simulink model "simulink2stopnie"  (R2024b)
settings: Solver=VariableStepAuto  StartTime=0.0  StopTime=10.0  RelTol=1e-3
values from neighbouring files (symbols this model uses):
  Amp = 1000    [stopnie_swobody.m]    (also in untitled.m)
  c1 = 10    [stopnie_swobody.m]    (also in untitled.m)
  c2 = 15    [stopnie_swobody.m]    (also in untitled.m)
  f = 10    [stopnie_swobody.m]    (also in untitled.m)
  k1 = 5000    [stopnie_swobody.m]    (also in untitled.m)
  k2 = 3000    [stopnie_swobody.m]    (also in untitled.m)
  m1 = 10    [stopnie_swobody.m]    (also in untitled.m)
  m2 = 15    [stopnie_swobody.m]    (also in untitled.m)
settings Model: Creator=jakub  LastModifiedBy=jakub

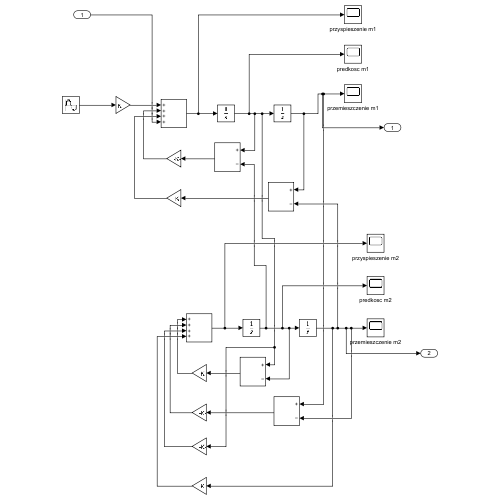
[thumbnail: Simulink's stored preview of the top-level diagram]
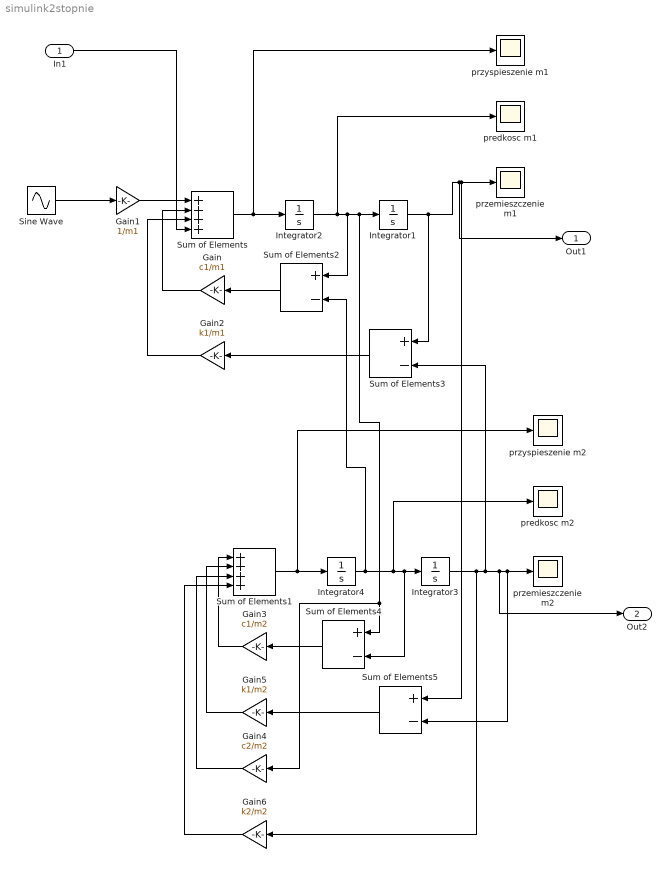
== system simulink2stopnie ==
  In1 : Inport
  Gain : Gain  Gain=c1/m1
  Gain1 : Gain  Gain=1/m1
  Gain2 : Gain  Gain=k1/m1
  Gain3 : Gain  Gain=c1/m2
  Gain4 : Gain  Gain=c2/m2
  Gain5 : Gain  Gain=k1/m2
  Gain6 : Gain  Gain=k2/m2
  Integrator{1..4} (4 alike) : Integrator
  Sine Wave : Sin  Amplitude=Amp  Frequency=2*pi*f  SampleTime=0.001
  Sum of Elements : Sum  Inputs=++++
  Sum of Elements1 : Sum  Inputs=++++
  Sum of Elements{2..5} (4 alike) : Sum  Inputs=+-
  predkosc m1 : Scope
  predkosc m2 : Scope
  przemieszczenie m1 : Scope
  przemieszczenie m2 : Scope
  przyspieszenie m1 : Scope
  przyspieszenie m2 : Scope
  Out1 : Outport
  Out2 : Outport  Port=2
  wires:
  Sine Wave/1 -> Gain1/1
  Gain1/1 -> Sum of Elements/1
  Integrator2/1 -> predkosc m1/1, Sum of Elements2/1, Gain4/1, Sum of Elements4/1, Integrator1/1
  Sum of Elements/1 -> przyspieszenie m1/1, Integrator2/1
  Gain/1 -> Sum of Elements/2
  Gain2/1 -> Sum of Elements/3
  In1/1 -> Sum of Elements/4
  Sum of Elements1/1 -> przyspieszenie m2/1, Integrator4/1
  Integrator4/1 -> predkosc m2/1, Sum of Elements4/2, Integrator3/1, Sum of Elements2/2
  Integrator3/1 -> Gain6/1, Sum of Elements3/2, Out2/1, Sum of Elements5/2, przemieszczenie m2/1
  Sum of Elements3/1 -> Gain2/1
  Integrator1/1 -> Sum of Elements3/1, przemieszczenie m1/1, Sum of Elements5/1, Out1/1
  Sum of Elements2/1 -> Gain/1
  Sum of Elements4/1 -> Gain3/1
  Sum of Elements5/1 -> Gain5/1
  Gain3/1 -> Sum of Elements1/1
  Gain5/1 -> Sum of Elements1/2
  Gain4/1 -> Sum of Elements1/3
  Gain6/1 -> Sum of Elements1/4
